simulink model "UDP_TEST"  (R2021a)
settings: Solver=VariableStepAuto  StartTime=0.0  StopTime=4  RelTol=1e-3
libraries: slrealtimeiplib x2
settings Model: Creator=olegg  LastModifiedBy=olegg

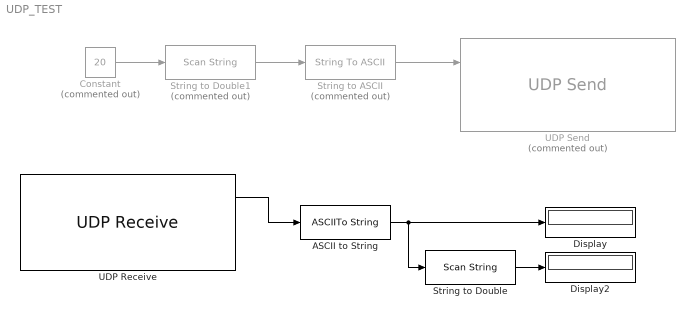
== system UDP_TEST ==
  ASCII to String : ASCIIToString
  Constant : Constant  Commented=on  Value=20
  Display : Display
  Display2 : Display
  String to ASCII : StringToASCII  Commented=on
  String to Double : ScanString  Format="\"%lf\""
  String to Double1 : ScanString  Commented=on  Format="\"%s\""
  UDP Receive : slrealtimeiplib/UDP Receive  useHostTargetConn=off  ipAddress=192.168.1.5  localPort=22  rcvWidth=16  rcvFmAny=off  fmAddress=192.168.1.11  sampleTime=10e-3
      settings: SourceProductBaseCode=XP
  UDP Send : slrealtimeiplib/UDP Send  Commented=on  useHostTargetConn=off  ipAddress=192.168.1.5  localPort=22  toAddress=192.168.1.11  toPort=11  sampleTime=1e-3
      settings: SourceProductBaseCode=XP
  wires:
  UDP Receive/1 -> ASCII to String/1
  ASCII to String/1 -> Display/1, String to Double/1
  String to Double/1 -> Display2/1
  Constant/1 -> String to Double1/1
  String to ASCII/1 -> UDP Send/1
  String to Double1/1 -> String to ASCII/1
